simulink model "ACC_Scenario_006_cs"  (R2014b)
settings: Solver=ode5  SolverMode=SingleTasking  StartTime=0.0  StopTime=inf  FixedStep=1/100  RelTol=1e-3
PreLoadFcn:
  | mbxruntime.callbacks.PreLoadFcn(bdroot);
  | check_NUTS_defined;
  | 
  | assignin('base',['model_closed_' bdroot],false);addpath('../includes_ACC');
PostLoadFcn:
  | mbxruntime.callbacks.PostLoadFcn(bdroot);
InitFcn:
  | mbxruntime.callbacks.InitFcn(bdroot);
StartFcn:
  | mbxruntime.callbacks.StartFcn(bdroot);
StopFcn:
  | mbxruntime.callbacks.StopFcn(bdroot);
model workspace: external: MAT-File .\ACC_Scenario_006_cs_hws.mat (data not in the file)
undefined symbols (not defined in the file or in its folder): mbxruntime, OrientationPitch, OrientationRoll, PositionX, PositionY, PositionZ, tabledata, warningInitialVelocity, x0
undefined symbols (not defined in the file): ACC_Scenario_006_cs_061450488d6753c4, ACC_Scenario_006_cs_13896134c615b72a, ACC_Scenario_006_cs_18eaf2a52f2ef75d, ACC_Scenario_006_cs_59e375456829d2f0, ACC_Scenario_006_cs_8a2109b915871f11, ACC_Scenario_006_cs_a4f79cab717c06e2, ACC_Scenario_006_cs_Audi_A8_1_Dynamics_Simple_initialPitch, ACC_Scenario_006_cs_Audi_A8_1_Dynamics_Simple_initialRoll, ACC_Scenario_006_cs_Audi_A8_1_Dynamics_Simple_initialX, ACC_Scenario_006_cs_Audi_A8_1_Dynamics_Simple_initialY, ACC_Scenario_006_cs_Audi_A8_1_Dynamics_Simple_initialYaw, ACC_Scenario_006_cs_Audi_A8_1_Dynamics_Simple_initialZ, ACC_Scenario_006_cs_BMW_X5_1_Path_pathUniqueID, ACC_Scenario_006_cs_BMW_X5_1_SpeedProfile_speedProfileUniqueID, ACC_Scenario_006_cs_e4633c18fd34a832, ACC_Scenario_006_cs_f83c81dc10cd364a, ACC_Scenario_006_cs_Fiat_Bravo_1_Path_pathUniqueID, ACC_Scenario_006_cs_Ford_Fiesta_1_Path_pathUniqueID, ACC_Scenario_006_cs_Honda_Pan_European_1_Path_pathUniqueID, ACC_Scenario_006_cs_Mazda_RX8_1_Path_pathUniqueID, ACC_Scenario_006_cs_Sphere_1_Dynamics_Empty_STATE_Sphere_1_x0, ACC_Scenario_006_cs_Sphere_1_Dynamics_Empty_STATE_Sphere_1_y0, ACC_Scenario_006_cs_Sphere_1_Dynamics_Empty_STATE_Sphere_1_Yaw0, ACC_Scenario_006_cs_Sphere_1_Dynamics_Empty_STATE_Sphere_1_z0, ACC_Scenario_006_cs_Toyota_Yaris_1_Path_pathUniqueID, SteeringColumn, SteeringWheel, Wheel0, Wheel0_Suspension, Wheel1, Wheel1_Suspension, WheelL0, WheelL1, WheelR0, WheelR1
libraries: simulink_extras x60, simulink x21, PreScanSimulinkLibrary x5, PreScanUsefulBlocks x2
(part 13 of 24)

== system ACC_Scenario_006_cs/HighwayOverhang_10/VISUMatrixSign_Mux ==
  InformationPlate_15 : Inport
  InformationPlate_16 : Inport  Port=2
  InformationPlate_15_Conversion : DataTypeConversion
  InformationPlate_15_InitialResource : Constant  Value=5
  InformationPlate_15_Switch : Switch  Criteria=u2 ~= 0
  InformationPlate_16_Conversion : DataTypeConversion
  InformationPlate_16_InitialResource : Constant  Value=5
  InformationPlate_16_Switch : Switch  Criteria=u2 ~= 0
  SubMuxMatrixSign : Mux  Inputs=2
  MatrixSigns : Outport
  wires:
  SubMuxMatrixSign/1 -> MatrixSigns/1
  InformationPlate_15/1 -> InformationPlate_15_Switch/1, InformationPlate_15_Switch/2
  InformationPlate_15_InitialResource/1 -> InformationPlate_15_Switch/3
  InformationPlate_15_Switch/1 -> InformationPlate_15_Conversion/1
  InformationPlate_15_Conversion/1 -> SubMuxMatrixSign/1
  InformationPlate_16/1 -> InformationPlate_16_Switch/1, InformationPlate_16_Switch/2
  InformationPlate_16_InitialResource/1 -> InformationPlate_16_Switch/3
  InformationPlate_16_Switch/1 -> InformationPlate_16_Conversion/1
  InformationPlate_16_Conversion/1 -> SubMuxMatrixSign/2

== system ACC_Scenario_006_cs/HighwayOverhang_11/VISUMatrixSignLights_Mux ==
  MatrixSign_7 : Inport  Tag=inport/MatrixSign_7  PortDimensions=4  SampleTime=1/100  BusOutputAsStruct=on
  MatrixSign_8 : Inport  Tag=inport/MatrixSign_8  Port=2  PortDimensions=4  SampleTime=1/100  BusOutputAsStruct=on
  MuxVisuLights : Mux  Inputs=2
  VISUMatrixSignLights_HighwayOverhang_11 : Outport  Tag=outport/VisuMatrixSignLights  SampleTime=1/100
  wires:
  MuxVisuLights/1 -> VISUMatrixSignLights_HighwayOverhang_11/1
  MatrixSign_7/1 -> MuxVisuLights/1
  MatrixSign_8/1 -> MuxVisuLights/2

== system ACC_Scenario_006_cs/HighwayOverhang_11/VISUMatrixSign_Mux ==
  MatrixSign_7 : Inport
  MatrixSign_8 : Inport  Port=2
  MatrixSign_7_Conversion : DataTypeConversion
  MatrixSign_7_InitialResource : Constant
  MatrixSign_7_Switch : Switch  Criteria=u2 ~= 0
  MatrixSign_8_Conversion : DataTypeConversion
  MatrixSign_8_InitialResource : Constant
  MatrixSign_8_Switch : Switch  Criteria=u2 ~= 0
  SubMuxMatrixSign : Mux  Inputs=2
  MatrixSigns : Outport
  wires:
  SubMuxMatrixSign/1 -> MatrixSigns/1
  MatrixSign_7/1 -> MatrixSign_7_Switch/1, MatrixSign_7_Switch/2
  MatrixSign_7_InitialResource/1 -> MatrixSign_7_Switch/3
  MatrixSign_7_Switch/1 -> MatrixSign_7_Conversion/1
  MatrixSign_7_Conversion/1 -> SubMuxMatrixSign/1
  MatrixSign_8/1 -> MatrixSign_8_Switch/1, MatrixSign_8_Switch/2
  MatrixSign_8_InitialResource/1 -> MatrixSign_8_Switch/3
  MatrixSign_8_Switch/1 -> MatrixSign_8_Conversion/1
  MatrixSign_8_Conversion/1 -> SubMuxMatrixSign/2

== system ACC_Scenario_006_cs/HighwayOverhang_12/VISUMatrixSignLights_Mux ==
  MatrixSign_5 : Inport  Tag=inport/MatrixSign_5  PortDimensions=4  SampleTime=1/100  BusOutputAsStruct=on
  MatrixSign_6 : Inport  Tag=inport/MatrixSign_6  Port=2  PortDimensions=4  SampleTime=1/100  BusOutputAsStruct=on
  MuxVisuLights : Mux  Inputs=2
  VISUMatrixSignLights_HighwayOverhang_12 : Outport  Tag=outport/VisuMatrixSignLights  SampleTime=1/100
  wires:
  MuxVisuLights/1 -> VISUMatrixSignLights_HighwayOverhang_12/1
  MatrixSign_5/1 -> MuxVisuLights/1
  MatrixSign_6/1 -> MuxVisuLights/2

== system ACC_Scenario_006_cs/HighwayOverhang_12/VISUMatrixSign_Mux ==
  MatrixSign_5 : Inport
  MatrixSign_6 : Inport  Port=2
  MatrixSign_5_Conversion : DataTypeConversion
  MatrixSign_5_InitialResource : Constant
  MatrixSign_5_Switch : Switch  Criteria=u2 ~= 0
  MatrixSign_6_Conversion : DataTypeConversion
  MatrixSign_6_InitialResource : Constant
  MatrixSign_6_Switch : Switch  Criteria=u2 ~= 0
  SubMuxMatrixSign : Mux  Inputs=2
  MatrixSigns : Outport
  wires:
  SubMuxMatrixSign/1 -> MatrixSigns/1
  MatrixSign_5/1 -> MatrixSign_5_Switch/1, MatrixSign_5_Switch/2
  MatrixSign_5_InitialResource/1 -> MatrixSign_5_Switch/3
  MatrixSign_5_Switch/1 -> MatrixSign_5_Conversion/1
  MatrixSign_5_Conversion/1 -> SubMuxMatrixSign/1
  MatrixSign_6/1 -> MatrixSign_6_Switch/1, MatrixSign_6_Switch/2
  MatrixSign_6_InitialResource/1 -> MatrixSign_6_Switch/3
  MatrixSign_6_Switch/1 -> MatrixSign_6_Conversion/1
  MatrixSign_6_Conversion/1 -> SubMuxMatrixSign/2

== system ACC_Scenario_006_cs/HighwayOverhang_2/VISUMatrixSignLights_Mux ==
  MatrixSign_3 : Inport  Tag=inport/MatrixSign_3  PortDimensions=4  SampleTime=1/100  BusOutputAsStruct=on
  MatrixSign_4 : Inport  Tag=inport/MatrixSign_4  Port=2  PortDimensions=4  SampleTime=1/100  BusOutputAsStruct=on
  MuxVisuLights : Mux  Inputs=2
  VISUMatrixSignLights_HighwayOverhang_2 : Outport  Tag=outport/VisuMatrixSignLights  SampleTime=1/100
  wires:
  MuxVisuLights/1 -> VISUMatrixSignLights_HighwayOverhang_2/1
  MatrixSign_3/1 -> MuxVisuLights/1
  MatrixSign_4/1 -> MuxVisuLights/2

== system ACC_Scenario_006_cs/HighwayOverhang_2/VISUMatrixSign_Mux ==
  MatrixSign_3 : Inport
  MatrixSign_4 : Inport  Port=2
  MatrixSign_3_Conversion : DataTypeConversion
  MatrixSign_3_InitialResource : Constant
  MatrixSign_3_Switch : Switch  Criteria=u2 ~= 0
  MatrixSign_4_Conversion : DataTypeConversion
  MatrixSign_4_InitialResource : Constant
  MatrixSign_4_Switch : Switch  Criteria=u2 ~= 0
  SubMuxMatrixSign : Mux  Inputs=2
  MatrixSigns : Outport
  wires:
  SubMuxMatrixSign/1 -> MatrixSigns/1
  MatrixSign_3/1 -> MatrixSign_3_Switch/1, MatrixSign_3_Switch/2
  MatrixSign_3_InitialResource/1 -> MatrixSign_3_Switch/3
  MatrixSign_3_Switch/1 -> MatrixSign_3_Conversion/1
  MatrixSign_3_Conversion/1 -> SubMuxMatrixSign/1
  MatrixSign_4/1 -> MatrixSign_4_Switch/1, MatrixSign_4_Switch/2
  MatrixSign_4_InitialResource/1 -> MatrixSign_4_Switch/3
  MatrixSign_4_Switch/1 -> MatrixSign_4_Conversion/1
  MatrixSign_4_Conversion/1 -> SubMuxMatrixSign/2

== system ACC_Scenario_006_cs/HighwayOverhang_3/VISUMatrixSign_Mux ==
  InformationPlate_1 : Inport
  InformationPlate_2 : Inport  Port=2
  InformationPlate_1_Conversion : DataTypeConversion
  InformationPlate_1_InitialResource : Constant  Value=2
  InformationPlate_1_Switch : Switch  Criteria=u2 ~= 0
  InformationPlate_2_Conversion : DataTypeConversion
  InformationPlate_2_InitialResource : Constant  Value=2
  InformationPlate_2_Switch : Switch  Criteria=u2 ~= 0
  SubMuxMatrixSign : Mux  Inputs=2
  MatrixSigns : Outport
  wires:
  SubMuxMatrixSign/1 -> MatrixSigns/1
  InformationPlate_1/1 -> InformationPlate_1_Switch/1, InformationPlate_1_Switch/2
  InformationPlate_1_InitialResource/1 -> InformationPlate_1_Switch/3
  InformationPlate_1_Switch/1 -> InformationPlate_1_Conversion/1
  InformationPlate_1_Conversion/1 -> SubMuxMatrixSign/1
  InformationPlate_2/1 -> InformationPlate_2_Switch/1, InformationPlate_2_Switch/2
  InformationPlate_2_InitialResource/1 -> InformationPlate_2_Switch/3
  InformationPlate_2_Switch/1 -> InformationPlate_2_Conversion/1
  InformationPlate_2_Conversion/1 -> SubMuxMatrixSign/2

== system ACC_Scenario_006_cs/HighwayOverhang_4/VISUMatrixSign_Mux ==
  InformationPlate_3 : Inport
  InformationPlate_4 : Inport  Port=2
  InformationPlate_3_Conversion : DataTypeConversion
  InformationPlate_3_InitialResource : Constant  Value=2
  InformationPlate_3_Switch : Switch  Criteria=u2 ~= 0
  InformationPlate_4_Conversion : DataTypeConversion
  InformationPlate_4_InitialResource : Constant  Value=2
  InformationPlate_4_Switch : Switch  Criteria=u2 ~= 0
  SubMuxMatrixSign : Mux  Inputs=2
  MatrixSigns : Outport
  wires:
  SubMuxMatrixSign/1 -> MatrixSigns/1
  InformationPlate_3/1 -> InformationPlate_3_Switch/1, InformationPlate_3_Switch/2
  InformationPlate_3_InitialResource/1 -> InformationPlate_3_Switch/3
  InformationPlate_3_Switch/1 -> InformationPlate_3_Conversion/1
  InformationPlate_3_Conversion/1 -> SubMuxMatrixSign/1
  InformationPlate_4/1 -> InformationPlate_4_Switch/1, InformationPlate_4_Switch/2
  InformationPlate_4_InitialResource/1 -> InformationPlate_4_Switch/3
  InformationPlate_4_Switch/1 -> InformationPlate_4_Conversion/1
  InformationPlate_4_Conversion/1 -> SubMuxMatrixSign/2

== system ACC_Scenario_006_cs/HighwayOverhang_5/VISUMatrixSign_Mux ==
  InformationPlate_5 : Inport
  InformationPlate_6 : Inport  Port=2
  InformationPlate_5_Conversion : DataTypeConversion
  InformationPlate_5_InitialResource : Constant  Value=3
  InformationPlate_5_Switch : Switch  Criteria=u2 ~= 0
  InformationPlate_6_Conversion : DataTypeConversion
  InformationPlate_6_InitialResource : Constant  Value=3
  InformationPlate_6_Switch : Switch  Criteria=u2 ~= 0
  SubMuxMatrixSign : Mux  Inputs=2
  MatrixSigns : Outport
  wires:
  SubMuxMatrixSign/1 -> MatrixSigns/1
  InformationPlate_5/1 -> InformationPlate_5_Switch/1, InformationPlate_5_Switch/2
  InformationPlate_5_InitialResource/1 -> InformationPlate_5_Switch/3
  InformationPlate_5_Switch/1 -> InformationPlate_5_Conversion/1
  InformationPlate_5_Conversion/1 -> SubMuxMatrixSign/1
  InformationPlate_6/1 -> InformationPlate_6_Switch/1, InformationPlate_6_Switch/2
  InformationPlate_6_InitialResource/1 -> InformationPlate_6_Switch/3
  InformationPlate_6_Switch/1 -> InformationPlate_6_Conversion/1
  InformationPlate_6_Conversion/1 -> SubMuxMatrixSign/2

== system ACC_Scenario_006_cs/HighwayOverhang_6/VISUMatrixSign_Mux ==
  InformationPlate_7 : Inport
  InformationPlate_8 : Inport  Port=2
  InformationPlate_7_Conversion : DataTypeConversion
  InformationPlate_7_InitialResource : Constant  Value=3
  InformationPlate_7_Switch : Switch  Criteria=u2 ~= 0
  InformationPlate_8_Conversion : DataTypeConversion
  InformationPlate_8_InitialResource : Constant  Value=3
  InformationPlate_8_Switch : Switch  Criteria=u2 ~= 0
  SubMuxMatrixSign : Mux  Inputs=2
  MatrixSigns : Outport
  wires:
  SubMuxMatrixSign/1 -> MatrixSigns/1
  InformationPlate_7/1 -> InformationPlate_7_Switch/1, InformationPlate_7_Switch/2
  InformationPlate_7_InitialResource/1 -> InformationPlate_7_Switch/3
  InformationPlate_7_Switch/1 -> InformationPlate_7_Conversion/1
  InformationPlate_7_Conversion/1 -> SubMuxMatrixSign/1
  InformationPlate_8/1 -> InformationPlate_8_Switch/1, InformationPlate_8_Switch/2
  InformationPlate_8_InitialResource/1 -> InformationPlate_8_Switch/3
  InformationPlate_8_Switch/1 -> InformationPlate_8_Conversion/1
  InformationPlate_8_Conversion/1 -> SubMuxMatrixSign/2

== system ACC_Scenario_006_cs/HighwayOverhang_7/VISUMatrixSign_Mux ==
  InformationPlate_9 : Inport
  InformationPlate_10 : Inport  Port=2
  InformationPlate_10_Conversion : DataTypeConversion
  InformationPlate_10_InitialResource : Constant  Value=4
  InformationPlate_10_Switch : Switch  Criteria=u2 ~= 0
  InformationPlate_9_Conversion : DataTypeConversion
  InformationPlate_9_InitialResource : Constant  Value=4
  InformationPlate_9_Switch : Switch  Criteria=u2 ~= 0
  SubMuxMatrixSign : Mux  Inputs=2
  MatrixSigns : Outport
  wires:
  SubMuxMatrixSign/1 -> MatrixSigns/1
  InformationPlate_9/1 -> InformationPlate_9_Switch/1, InformationPlate_9_Switch/2
  InformationPlate_9_InitialResource/1 -> InformationPlate_9_Switch/3
  InformationPlate_9_Switch/1 -> InformationPlate_9_Conversion/1
  InformationPlate_9_Conversion/1 -> SubMuxMatrixSign/1
  InformationPlate_10/1 -> InformationPlate_10_Switch/1, InformationPlate_10_Switch/2
  InformationPlate_10_InitialResource/1 -> InformationPlate_10_Switch/3
  InformationPlate_10_Switch/1 -> InformationPlate_10_Conversion/1
  InformationPlate_10_Conversion/1 -> SubMuxMatrixSign/2

== system ACC_Scenario_006_cs/HighwayOverhang_8/VISUMatrixSign_Mux ==
  InformationPlate_11 : Inport
  InformationPlate_12 : Inport  Port=2
  InformationPlate_11_Conversion : DataTypeConversion
  InformationPlate_11_InitialResource : Constant  Value=4
  InformationPlate_11_Switch : Switch  Criteria=u2 ~= 0
  InformationPlate_12_Conversion : DataTypeConversion
  InformationPlate_12_InitialResource : Constant  Value=4
  InformationPlate_12_Switch : Switch  Criteria=u2 ~= 0
  SubMuxMatrixSign : Mux  Inputs=2
  MatrixSigns : Outport
  wires:
  SubMuxMatrixSign/1 -> MatrixSigns/1
  InformationPlate_11/1 -> InformationPlate_11_Switch/1, InformationPlate_11_Switch/2
  InformationPlate_11_InitialResource/1 -> InformationPlate_11_Switch/3
  InformationPlate_11_Switch/1 -> InformationPlate_11_Conversion/1
  InformationPlate_11_Conversion/1 -> SubMuxMatrixSign/1
  InformationPlate_12/1 -> InformationPlate_12_Switch/1, InformationPlate_12_Switch/2
  InformationPlate_12_InitialResource/1 -> InformationPlate_12_Switch/3
  InformationPlate_12_Switch/1 -> InformationPlate_12_Conversion/1
  InformationPlate_12_Conversion/1 -> SubMuxMatrixSign/2

== system ACC_Scenario_006_cs/HighwayOverhang_9/VISUMatrixSign_Mux ==
  InformationPlate_13 : Inport
  InformationPlate_14 : Inport  Port=2
  InformationPlate_13_Conversion : DataTypeConversion
  InformationPlate_13_InitialResource : Constant  Value=5
  InformationPlate_13_Switch : Switch  Criteria=u2 ~= 0
  InformationPlate_14_Conversion : DataTypeConversion
  InformationPlate_14_InitialResource : Constant  Value=5
  InformationPlate_14_Switch : Switch  Criteria=u2 ~= 0
  SubMuxMatrixSign : Mux  Inputs=2
  MatrixSigns : Outport
  wires:
  SubMuxMatrixSign/1 -> MatrixSigns/1
  InformationPlate_13/1 -> InformationPlate_13_Switch/1, InformationPlate_13_Switch/2
  InformationPlate_13_InitialResource/1 -> InformationPlate_13_Switch/3
  InformationPlate_13_Switch/1 -> InformationPlate_13_Conversion/1
  InformationPlate_13_Conversion/1 -> SubMuxMatrixSign/1
  InformationPlate_14/1 -> InformationPlate_14_Switch/1, InformationPlate_14_Switch/2
  InformationPlate_14_InitialResource/1 -> InformationPlate_14_Switch/3
  InformationPlate_14_Switch/1 -> InformationPlate_14_Conversion/1
  InformationPlate_14_Conversion/1 -> SubMuxMatrixSign/2

== system ACC_Scenario_006_cs/Honda_Pan_European_1/Brake_light_center_Mux ==
  MSCD [Cd] : Inport
  Position (xyz) [m] : Inport  Port=2
  Orientation (RPY) [deg] : Inport  Port=3
  Color [-] : Inport  Port=4
  TextureResourceID [-] : Inport  Port=5
  Bus Creator : BusCreator  Inputs='Intensity','Position','Orientation','Color','TextureResourceID'  OutDataTypeStr=Bus: PRESCAN_VISULIGHTACTUATOR_DATA  NonVirtualBus=on
  Bus Creator1 : BusCreator  Inputs=3  OutDataTypeStr=Bus: PRESCAN_RGB_DATA  NonVirtualBus=on
  Bus Creator2 : BusCreator  Inputs=3  OutDataTypeStr=Bus: PRESCAN_RPY_DATA  NonVirtualBus=on
  Bus Creator3 : BusCreator  Inputs=3  OutDataTypeStr=Bus: PRESCAN_XYZ_DATA  NonVirtualBus=on
  Data Type Conversion : DataTypeConversion  OutDataTypeStr=int32  RndMeth=Nearest
  Degrees to Radians : simulink_extras/Transformations/Degrees to Radians
  Demux : Demux  Outputs=3
  Demux1 : Demux  Outputs=3
  Demux2 : Demux  Outputs=3
  Lights : Outport
  wires:
  TextureResourceID [-]/1 -> Data Type Conversion/1  "TextureResourceID"
  MSCD [Cd]/1 -> Bus Creator/1  "Intensity"
  Bus Creator/1 -> Lights/1
  Demux/1 -> Bus Creator1/1  "R"
  Demux/2 -> Bus Creator1/2  "G"
  Demux/3 -> Bus Creator1/3  "B"
  Color [-]/1 -> Demux/1  "Color"
  Bus Creator1/1 -> Bus Creator/4  "Color"
  Demux1/1 -> Bus Creator2/1  "Roll"
  Demux1/2 -> Bus Creator2/2  "Pitch"
  Demux1/3 -> Bus Creator2/3  "Yaw"
  Orientation (RPY) [deg]/1 -> Degrees to Radians/1  "Orientation"
  Bus Creator2/1 -> Bus Creator/3  "Orientation"
  Demux2/1 -> Bus Creator3/1  "X"
  Demux2/2 -> Bus Creator3/2  "Y"
  Demux2/3 -> Bus Creator3/3  "Z"
  Position (xyz) [m]/1 -> Demux2/1  "Position"
  Bus Creator3/1 -> Bus Creator/2  "Position"
  Data Type Conversion/1 -> Bus Creator/5  "TextureResourceID"
  Degrees to Radians/1 -> Demux1/1

== system ACC_Scenario_006_cs/Honda_Pan_European_1/Indicator_front_left_Mux ==
  MSCD [Cd] : Inport
  Position (xyz) [m] : Inport  Port=2
  Orientation (RPY) [deg] : Inport  Port=3
  Color [-] : Inport  Port=4
  TextureResourceID [-] : Inport  Port=5
  Bus Creator : BusCreator  Inputs='Intensity','Position','Orientation','Color','TextureResourceID'  OutDataTypeStr=Bus: PRESCAN_VISULIGHTACTUATOR_DATA  NonVirtualBus=on
  Bus Creator1 : BusCreator  Inputs=3  OutDataTypeStr=Bus: PRESCAN_RGB_DATA  NonVirtualBus=on
  Bus Creator2 : BusCreator  Inputs=3  OutDataTypeStr=Bus: PRESCAN_RPY_DATA  NonVirtualBus=on
  Bus Creator3 : BusCreator  Inputs=3  OutDataTypeStr=Bus: PRESCAN_XYZ_DATA  NonVirtualBus=on
  Data Type Conversion : DataTypeConversion  OutDataTypeStr=int32  RndMeth=Nearest
  Degrees to Radians : simulink_extras/Transformations/Degrees to Radians
  Demux : Demux  Outputs=3
  Demux1 : Demux  Outputs=3
  Demux2 : Demux  Outputs=3
  Lights : Outport
  wires:
  TextureResourceID [-]/1 -> Data Type Conversion/1  "TextureResourceID"
  MSCD [Cd]/1 -> Bus Creator/1  "Intensity"
  Bus Creator/1 -> Lights/1
  Demux/1 -> Bus Creator1/1  "R"
  Demux/2 -> Bus Creator1/2  "G"
  Demux/3 -> Bus Creator1/3  "B"
  Color [-]/1 -> Demux/1  "Color"
  Bus Creator1/1 -> Bus Creator/4  "Color"
  Demux1/1 -> Bus Creator2/1  "Roll"
  Demux1/2 -> Bus Creator2/2  "Pitch"
  Demux1/3 -> Bus Creator2/3  "Yaw"
  Orientation (RPY) [deg]/1 -> Degrees to Radians/1  "Orientation"
  Bus Creator2/1 -> Bus Creator/3  "Orientation"
  Demux2/1 -> Bus Creator3/1  "X"
  Demux2/2 -> Bus Creator3/2  "Y"
  Demux2/3 -> Bus Creator3/3  "Z"
  Position (xyz) [m]/1 -> Demux2/1  "Position"
  Bus Creator3/1 -> Bus Creator/2  "Position"
  Data Type Conversion/1 -> Bus Creator/5  "TextureResourceID"
  Degrees to Radians/1 -> Demux1/1

== system ACC_Scenario_006_cs/Honda_Pan_European_1/Indicator_front_right_Mux ==
  MSCD [Cd] : Inport
  Position (xyz) [m] : Inport  Port=2
  Orientation (RPY) [deg] : Inport  Port=3
  Color [-] : Inport  Port=4
  TextureResourceID [-] : Inport  Port=5
  Bus Creator : BusCreator  Inputs='Intensity','Position','Orientation','Color','TextureResourceID'  OutDataTypeStr=Bus: PRESCAN_VISULIGHTACTUATOR_DATA  NonVirtualBus=on
  Bus Creator1 : BusCreator  Inputs=3  OutDataTypeStr=Bus: PRESCAN_RGB_DATA  NonVirtualBus=on
  Bus Creator2 : BusCreator  Inputs=3  OutDataTypeStr=Bus: PRESCAN_RPY_DATA  NonVirtualBus=on
  Bus Creator3 : BusCreator  Inputs=3  OutDataTypeStr=Bus: PRESCAN_XYZ_DATA  NonVirtualBus=on
  Data Type Conversion : DataTypeConversion  OutDataTypeStr=int32  RndMeth=Nearest
  Degrees to Radians : simulink_extras/Transformations/Degrees to Radians
  Demux : Demux  Outputs=3
  Demux1 : Demux  Outputs=3
  Demux2 : Demux  Outputs=3
  Lights : Outport
  wires:
  TextureResourceID [-]/1 -> Data Type Conversion/1  "TextureResourceID"
  MSCD [Cd]/1 -> Bus Creator/1  "Intensity"
  Bus Creator/1 -> Lights/1
  Demux/1 -> Bus Creator1/1  "R"
  Demux/2 -> Bus Creator1/2  "G"
  Demux/3 -> Bus Creator1/3  "B"
  Color [-]/1 -> Demux/1  "Color"
  Bus Creator1/1 -> Bus Creator/4  "Color"
  Demux1/1 -> Bus Creator2/1  "Roll"
  Demux1/2 -> Bus Creator2/2  "Pitch"
  Demux1/3 -> Bus Creator2/3  "Yaw"
  Orientation (RPY) [deg]/1 -> Degrees to Radians/1  "Orientation"
  Bus Creator2/1 -> Bus Creator/3  "Orientation"
  Demux2/1 -> Bus Creator3/1  "X"
  Demux2/2 -> Bus Creator3/2  "Y"
  Demux2/3 -> Bus Creator3/3  "Z"
  Position (xyz) [m]/1 -> Demux2/1  "Position"
  Bus Creator3/1 -> Bus Creator/2  "Position"
  Data Type Conversion/1 -> Bus Creator/5  "TextureResourceID"
  Degrees to Radians/1 -> Demux1/1

== system ACC_Scenario_006_cs/Honda_Pan_European_1/Indicator_rear_left_Mux ==
  MSCD [Cd] : Inport
  Position (xyz) [m] : Inport  Port=2
  Orientation (RPY) [deg] : Inport  Port=3
  Color [-] : Inport  Port=4
  TextureResourceID [-] : Inport  Port=5
  Bus Creator : BusCreator  Inputs='Intensity','Position','Orientation','Color','TextureResourceID'  OutDataTypeStr=Bus: PRESCAN_VISULIGHTACTUATOR_DATA  NonVirtualBus=on
  Bus Creator1 : BusCreator  Inputs=3  OutDataTypeStr=Bus: PRESCAN_RGB_DATA  NonVirtualBus=on
  Bus Creator2 : BusCreator  Inputs=3  OutDataTypeStr=Bus: PRESCAN_RPY_DATA  NonVirtualBus=on
  Bus Creator3 : BusCreator  Inputs=3  OutDataTypeStr=Bus: PRESCAN_XYZ_DATA  NonVirtualBus=on
  Data Type Conversion : DataTypeConversion  OutDataTypeStr=int32  RndMeth=Nearest
  Degrees to Radians : simulink_extras/Transformations/Degrees to Radians
  Demux : Demux  Outputs=3
  Demux1 : Demux  Outputs=3
  Demux2 : Demux  Outputs=3
  Lights : Outport
  wires:
  TextureResourceID [-]/1 -> Data Type Conversion/1  "TextureResourceID"
  MSCD [Cd]/1 -> Bus Creator/1  "Intensity"
  Bus Creator/1 -> Lights/1
  Demux/1 -> Bus Creator1/1  "R"
  Demux/2 -> Bus Creator1/2  "G"
  Demux/3 -> Bus Creator1/3  "B"
  Color [-]/1 -> Demux/1  "Color"
  Bus Creator1/1 -> Bus Creator/4  "Color"
  Demux1/1 -> Bus Creator2/1  "Roll"
  Demux1/2 -> Bus Creator2/2  "Pitch"
  Demux1/3 -> Bus Creator2/3  "Yaw"
  Orientation (RPY) [deg]/1 -> Degrees to Radians/1  "Orientation"
  Bus Creator2/1 -> Bus Creator/3  "Orientation"
  Demux2/1 -> Bus Creator3/1  "X"
  Demux2/2 -> Bus Creator3/2  "Y"
  Demux2/3 -> Bus Creator3/3  "Z"
  Position (xyz) [m]/1 -> Demux2/1  "Position"
  Bus Creator3/1 -> Bus Creator/2  "Position"
  Data Type Conversion/1 -> Bus Creator/5  "TextureResourceID"
  Degrees to Radians/1 -> Demux1/1

== system ACC_Scenario_006_cs/Honda_Pan_European_1/Indicator_rear_right_Mux ==
  MSCD [Cd] : Inport
  Position (xyz) [m] : Inport  Port=2
  Orientation (RPY) [deg] : Inport  Port=3
  Color [-] : Inport  Port=4
  TextureResourceID [-] : Inport  Port=5
  Bus Creator : BusCreator  Inputs='Intensity','Position','Orientation','Color','TextureResourceID'  OutDataTypeStr=Bus: PRESCAN_VISULIGHTACTUATOR_DATA  NonVirtualBus=on
  Bus Creator1 : BusCreator  Inputs=3  OutDataTypeStr=Bus: PRESCAN_RGB_DATA  NonVirtualBus=on
  Bus Creator2 : BusCreator  Inputs=3  OutDataTypeStr=Bus: PRESCAN_RPY_DATA  NonVirtualBus=on
  Bus Creator3 : BusCreator  Inputs=3  OutDataTypeStr=Bus: PRESCAN_XYZ_DATA  NonVirtualBus=on
  Data Type Conversion : DataTypeConversion  OutDataTypeStr=int32  RndMeth=Nearest
  Degrees to Radians : simulink_extras/Transformations/Degrees to Radians
  Demux : Demux  Outputs=3
  Demux1 : Demux  Outputs=3
  Demux2 : Demux  Outputs=3
  Lights : Outport
  wires:
  TextureResourceID [-]/1 -> Data Type Conversion/1  "TextureResourceID"
  MSCD [Cd]/1 -> Bus Creator/1  "Intensity"
  Bus Creator/1 -> Lights/1
  Demux/1 -> Bus Creator1/1  "R"
  Demux/2 -> Bus Creator1/2  "G"
  Demux/3 -> Bus Creator1/3  "B"
  Color [-]/1 -> Demux/1  "Color"
  Bus Creator1/1 -> Bus Creator/4  "Color"
  Demux1/1 -> Bus Creator2/1  "Roll"
  Demux1/2 -> Bus Creator2/2  "Pitch"
  Demux1/3 -> Bus Creator2/3  "Yaw"
  Orientation (RPY) [deg]/1 -> Degrees to Radians/1  "Orientation"
  Bus Creator2/1 -> Bus Creator/3  "Orientation"
  Demux2/1 -> Bus Creator3/1  "X"
  Demux2/2 -> Bus Creator3/2  "Y"
  Demux2/3 -> Bus Creator3/3  "Z"
  Position (xyz) [m]/1 -> Demux2/1  "Position"
  Bus Creator3/1 -> Bus Creator/2  "Position"
  Data Type Conversion/1 -> Bus Creator/5  "TextureResourceID"
  Degrees to Radians/1 -> Demux1/1

== system ACC_Scenario_006_cs/Honda_Pan_European_1/SELF_Demux ==
  SELF : Inport  OutDataTypeStr=Bus: PRESCAN_SELFSENSORDATA
  Bus Selector : BusSelector  OutputSignals=PositionX,PositionY,PositionZ,OrientationRoll,OrientationPitch,OrientationYaw,Velocity,Yaw_rate,Lat,Long,Alt
  Demux2 : Demux  Outputs=3
  Gain : Gain  Gain=180/pi
  Gain1 : Gain  Gain=180/pi
  Vector Concatenate1 : Concatenate  NumInputs=3
  compas converter : Subsystem
  x [m] : Outport
  y [m] : Outport  Port=2
  z [m] : Outport  Port=3
  rotx [deg] : Outport  Port=4
  roty [deg] : Outport  Port=5
  rotz [deg] : Outport  Port=6
  GPS lat [deg] : Outport  Port=7
  GPS long [deg] : Outport  Port=8
  GPS alt [m] : Outport  Port=9
  velocity [m/s] : Outport  Port=10
  heading [deg] : Outport  Port=11
  yaw rate [deg/s] : Outport  Port=12
  wires:
  Bus Selector/11 -> GPS alt [m]/1  "<Alt>"
  Bus Selector/10 -> GPS long [deg]/1  "<Long>"
  Bus Selector/9 -> GPS lat [deg]/1  "<Lat>"
  Bus Selector/8 -> Gain1/1  "<Yaw_rate>"
  Bus Selector/7 -> velocity [m/s]/1  "<Velocity>"
  Bus Selector/6 -> compas converter/1(rotz [rad]), Vector Concatenate1/3  "<OrientationYaw>"
  Bus Selector/5 -> Vector Concatenate1/2  "<OrientationPitch>"
  Bus Selector/4 -> Vector Concatenate1/1  "<OrientationRoll>"
  Vector Concatenate1/1 -> Gain/1
  Bus Selector/3 -> z [m]/1  "<PositionZ>"
  Bus Selector/2 -> y [m]/1  "<PositionY>"
  Bus Selector/1 -> x [m]/1  "<PositionX>"
  SELF/1 -> Bus Selector/1
  Gain/1 -> Demux2/1
  Demux2/1 -> rotx [deg]/1
  Demux2/2 -> roty [deg]/1
  Demux2/3 -> rotz [deg]/1
  compas converter/1(heading [deg]) -> heading [deg]/1
  Gain1/1 -> yaw rate [deg/s]/1

== system ACC_Scenario_006_cs/Honda_Pan_European_1/V2R_WheelMC ==
  Velocity [m/s] : Inport  SampleTime=TimeStep
  Discrete-Time Integrator : DiscreteIntegrator  SampleTime=TimeStep
  omega=V/Rwheel : Gain  Gain=1/TireRadius
  Rotation [rad] : Outport
  wires:
  Velocity [m/s]/1 -> omega=V/Rwheel/1
  omega=V/Rwheel/1 -> Discrete-Time Integrator/1  "rotational speed [rad/s]"
  Discrete-Time Integrator/1 -> Rotation [rad]/1  "roty"

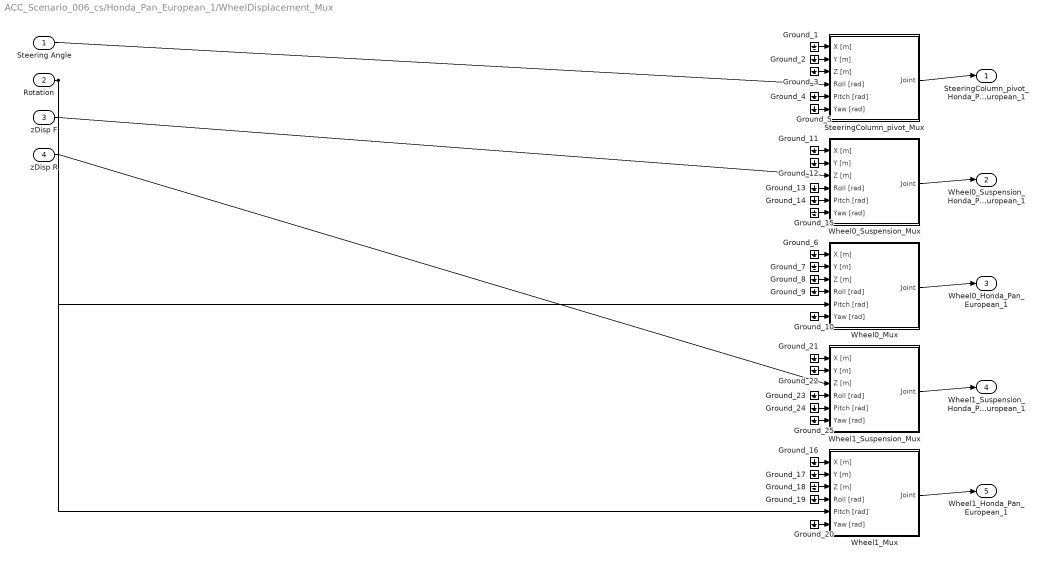
== system ACC_Scenario_006_cs/Honda_Pan_European_1/WheelDisplacement_Mux ==
  Steering Angle : Inport  Tag=inport/JointGroup  SampleTime=1/100  BusOutputAsStruct=on
  Rotation : Inport  Tag=inport/JointGroup  Port=2  SampleTime=1/100  BusOutputAsStruct=on
  zDisp F : Inport  Tag=inport/JointGroup  Port=3  SampleTime=1/100  BusOutputAsStruct=on
  zDisp R : Inport  Tag=inport/JointGroup  Port=4  SampleTime=1/100  BusOutputAsStruct=on
  Ground_{1..25} (25 alike) : Ground
  SteeringColumn_pivot_Mux : Subsystem  Tag=mux/Joint  mask(PreScan Mux Block){DisplayName=SteeringColumn}
      mask prompts: DisplayName "Display Name"
      mask help:
      | This block simulates a generic joint used for generic models. This joint can be enabled/disabled from the GUI.
      |
      | For more information, please click Help.
      settings: DeleteFcn=PreScanBlockDeleteFcn;
      mask Help: eval('openHelp(254)')
  Wheel0_Mux : Subsystem  Tag=mux/Joint  mask(PreScan Mux Block){DisplayName=Wheel0}
      mask prompts: DisplayName "Display Name"
      mask help:
      | This block simulates a generic joint used for generic models. This joint can be enabled/disabled from the GUI.
      |
      | For more information, please click Help.
      settings: DeleteFcn=PreScanBlockDeleteFcn;
      mask Help: eval('openHelp(254)')
  Wheel0_Suspension_Mux : Subsystem  Tag=mux/Joint  mask(PreScan Mux Block){DisplayName=Wheel0_Suspension}
      mask prompts: DisplayName "Display Name"
      mask help:
      | This block simulates a generic joint used for generic models. This joint can be enabled/disabled from the GUI.
      |
      | For more information, please click Help.
      settings: DeleteFcn=PreScanBlockDeleteFcn;
      mask Help: eval('openHelp(254)')
  Wheel1_Mux : Subsystem  Tag=mux/Joint  mask(PreScan Mux Block){DisplayName=Wheel1}
      mask prompts: DisplayName "Display Name"
      mask help:
      | This block simulates a generic joint used for generic models. This joint can be enabled/disabled from the GUI.
      |
      | For more information, please click Help.
      settings: DeleteFcn=PreScanBlockDeleteFcn;
      mask Help: eval('openHelp(254)')
  Wheel1_Suspension_Mux : Subsystem  Tag=mux/Joint  mask(PreScan Mux Block){DisplayName=Wheel1_Suspension}
      mask prompts: DisplayName "Display Name"
      mask help:
      | This block simulates a generic joint used for generic models. This joint can be enabled/disabled from the GUI.
      |
      | For more information, please click Help.
      settings: DeleteFcn=PreScanBlockDeleteFcn;
      mask Help: eval('openHelp(254)')
  SteeringColumn_pivot_Honda_Pan_European_1 : Outport  Tag=outport/JointActuator  OutDataTypeStr=Bus: PRESCAN_POSE_DATA  SampleTime=1/100
  Wheel0_Suspension_Honda_Pan_European_1 : Outport  Tag=outport/JointActuator  Port=2  OutDataTypeStr=Bus: PRESCAN_POSE_DATA  SampleTime=1/100
  Wheel0_Honda_Pan_European_1 : Outport  Tag=outport/JointActuator  Port=3  OutDataTypeStr=Bus: PRESCAN_POSE_DATA  SampleTime=1/100
  Wheel1_Suspension_Honda_Pan_European_1 : Outport  Tag=outport/JointActuator  Port=4  OutDataTypeStr=Bus: PRESCAN_POSE_DATA  SampleTime=1/100
  Wheel1_Honda_Pan_European_1 : Outport  Tag=outport/JointActuator  Port=5  OutDataTypeStr=Bus: PRESCAN_POSE_DATA  SampleTime=1/100
  wires:
  SteeringColumn_pivot_Mux/1(Joint) -> SteeringColumn_pivot_Honda_Pan_European_1/1
  Wheel0_Suspension_Mux/1(Joint) -> Wheel0_Suspension_Honda_Pan_European_1/1
  Wheel0_Mux/1(Joint) -> Wheel0_Honda_Pan_European_1/1
  Wheel1_Suspension_Mux/1(Joint) -> Wheel1_Suspension_Honda_Pan_European_1/1
  Wheel1_Mux/1(Joint) -> Wheel1_Honda_Pan_European_1/1
  Steering Angle/1 -> SteeringColumn_pivot_Mux/4(Roll [rad])
  Rotation/1 -> Wheel0_Mux/5(Pitch [rad]), Wheel1_Mux/5(Pitch [rad])
  zDisp F/1 -> Wheel0_Suspension_Mux/3(Z [m])
  zDisp R/1 -> Wheel1_Suspension_Mux/3(Z [m])
  Ground_1/1 -> SteeringColumn_pivot_Mux/1(X [m])
  Ground_2/1 -> SteeringColumn_pivot_Mux/2(Y [m])
  Ground_3/1 -> SteeringColumn_pivot_Mux/3(Z [m])
  Ground_4/1 -> SteeringColumn_pivot_Mux/5(Pitch [rad])
  Ground_5/1 -> SteeringColumn_pivot_Mux/6(Yaw [rad])
  Ground_6/1 -> Wheel0_Mux/1(X [m])
  Ground_7/1 -> Wheel0_Mux/2(Y [m])
  Ground_8/1 -> Wheel0_Mux/3(Z [m])
  Ground_9/1 -> Wheel0_Mux/4(Roll [rad])
  Ground_10/1 -> Wheel0_Mux/6(Yaw [rad])
  Ground_11/1 -> Wheel0_Suspension_Mux/1(X [m])
  Ground_12/1 -> Wheel0_Suspension_Mux/2(Y [m])
  Ground_13/1 -> Wheel0_Suspension_Mux/4(Roll [rad])
  Ground_14/1 -> Wheel0_Suspension_Mux/5(Pitch [rad])
  Ground_15/1 -> Wheel0_Suspension_Mux/6(Yaw [rad])
  Ground_16/1 -> Wheel1_Mux/1(X [m])
  Ground_17/1 -> Wheel1_Mux/2(Y [m])
  Ground_18/1 -> Wheel1_Mux/3(Z [m])
  Ground_19/1 -> Wheel1_Mux/4(Roll [rad])
  Ground_20/1 -> Wheel1_Mux/6(Yaw [rad])
  Ground_21/1 -> Wheel1_Suspension_Mux/1(X [m])
  Ground_22/1 -> Wheel1_Suspension_Mux/2(Y [m])
  Ground_23/1 -> Wheel1_Suspension_Mux/4(Roll [rad])
  Ground_24/1 -> Wheel1_Suspension_Mux/5(Pitch [rad])
  Ground_25/1 -> Wheel1_Suspension_Mux/6(Yaw [rad])

== system ACC_Scenario_006_cs/Mazda_RX8_1/Brake_light_center_Mux ==
  MSCD [Cd] : Inport
  Position (xyz) [m] : Inport  Port=2
  Orientation (RPY) [deg] : Inport  Port=3
  Color [-] : Inport  Port=4
  TextureResourceID [-] : Inport  Port=5
  Bus Creator : BusCreator  Inputs='Intensity','Position','Orientation','Color','TextureResourceID'  OutDataTypeStr=Bus: PRESCAN_VISULIGHTACTUATOR_DATA  NonVirtualBus=on
  Bus Creator1 : BusCreator  Inputs=3  OutDataTypeStr=Bus: PRESCAN_RGB_DATA  NonVirtualBus=on
  Bus Creator2 : BusCreator  Inputs=3  OutDataTypeStr=Bus: PRESCAN_RPY_DATA  NonVirtualBus=on
  Bus Creator3 : BusCreator  Inputs=3  OutDataTypeStr=Bus: PRESCAN_XYZ_DATA  NonVirtualBus=on
  Data Type Conversion : DataTypeConversion  OutDataTypeStr=int32  RndMeth=Nearest
  Degrees to Radians : simulink_extras/Transformations/Degrees to Radians
  Demux : Demux  Outputs=3
  Demux1 : Demux  Outputs=3
  Demux2 : Demux  Outputs=3
  Lights : Outport
  wires:
  TextureResourceID [-]/1 -> Data Type Conversion/1  "TextureResourceID"
  MSCD [Cd]/1 -> Bus Creator/1  "Intensity"
  Bus Creator/1 -> Lights/1
  Demux/1 -> Bus Creator1/1  "R"
  Demux/2 -> Bus Creator1/2  "G"
  Demux/3 -> Bus Creator1/3  "B"
  Color [-]/1 -> Demux/1  "Color"
  Bus Creator1/1 -> Bus Creator/4  "Color"
  Demux1/1 -> Bus Creator2/1  "Roll"
  Demux1/2 -> Bus Creator2/2  "Pitch"
  Demux1/3 -> Bus Creator2/3  "Yaw"
  Orientation (RPY) [deg]/1 -> Degrees to Radians/1  "Orientation"
  Bus Creator2/1 -> Bus Creator/3  "Orientation"
  Demux2/1 -> Bus Creator3/1  "X"
  Demux2/2 -> Bus Creator3/2  "Y"
  Demux2/3 -> Bus Creator3/3  "Z"
  Position (xyz) [m]/1 -> Demux2/1  "Position"
  Bus Creator3/1 -> Bus Creator/2  "Position"
  Data Type Conversion/1 -> Bus Creator/5  "TextureResourceID"
  Degrees to Radians/1 -> Demux1/1

== system ACC_Scenario_006_cs/Mazda_RX8_1/Brake_light_left_Mux ==
  MSCD [Cd] : Inport
  Position (xyz) [m] : Inport  Port=2
  Orientation (RPY) [deg] : Inport  Port=3
  Color [-] : Inport  Port=4
  TextureResourceID [-] : Inport  Port=5
  Bus Creator : BusCreator  Inputs='Intensity','Position','Orientation','Color','TextureResourceID'  OutDataTypeStr=Bus: PRESCAN_VISULIGHTACTUATOR_DATA  NonVirtualBus=on
  Bus Creator1 : BusCreator  Inputs=3  OutDataTypeStr=Bus: PRESCAN_RGB_DATA  NonVirtualBus=on
  Bus Creator2 : BusCreator  Inputs=3  OutDataTypeStr=Bus: PRESCAN_RPY_DATA  NonVirtualBus=on
  Bus Creator3 : BusCreator  Inputs=3  OutDataTypeStr=Bus: PRESCAN_XYZ_DATA  NonVirtualBus=on
  Data Type Conversion : DataTypeConversion  OutDataTypeStr=int32  RndMeth=Nearest
  Degrees to Radians : simulink_extras/Transformations/Degrees to Radians
  Demux : Demux  Outputs=3
  Demux1 : Demux  Outputs=3
  Demux2 : Demux  Outputs=3
  Lights : Outport
  wires:
  TextureResourceID [-]/1 -> Data Type Conversion/1  "TextureResourceID"
  MSCD [Cd]/1 -> Bus Creator/1  "Intensity"
  Bus Creator/1 -> Lights/1
  Demux/1 -> Bus Creator1/1  "R"
  Demux/2 -> Bus Creator1/2  "G"
  Demux/3 -> Bus Creator1/3  "B"
  Color [-]/1 -> Demux/1  "Color"
  Bus Creator1/1 -> Bus Creator/4  "Color"
  Demux1/1 -> Bus Creator2/1  "Roll"
  Demux1/2 -> Bus Creator2/2  "Pitch"
  Demux1/3 -> Bus Creator2/3  "Yaw"
  Orientation (RPY) [deg]/1 -> Degrees to Radians/1  "Orientation"
  Bus Creator2/1 -> Bus Creator/3  "Orientation"
  Demux2/1 -> Bus Creator3/1  "X"
  Demux2/2 -> Bus Creator3/2  "Y"
  Demux2/3 -> Bus Creator3/3  "Z"
  Position (xyz) [m]/1 -> Demux2/1  "Position"
  Bus Creator3/1 -> Bus Creator/2  "Position"
  Data Type Conversion/1 -> Bus Creator/5  "TextureResourceID"
  Degrees to Radians/1 -> Demux1/1

== system ACC_Scenario_006_cs/Mazda_RX8_1/Brake_light_right_Mux ==
  MSCD [Cd] : Inport
  Position (xyz) [m] : Inport  Port=2
  Orientation (RPY) [deg] : Inport  Port=3
  Color [-] : Inport  Port=4
  TextureResourceID [-] : Inport  Port=5
  Bus Creator : BusCreator  Inputs='Intensity','Position','Orientation','Color','TextureResourceID'  OutDataTypeStr=Bus: PRESCAN_VISULIGHTACTUATOR_DATA  NonVirtualBus=on
  Bus Creator1 : BusCreator  Inputs=3  OutDataTypeStr=Bus: PRESCAN_RGB_DATA  NonVirtualBus=on
  Bus Creator2 : BusCreator  Inputs=3  OutDataTypeStr=Bus: PRESCAN_RPY_DATA  NonVirtualBus=on
  Bus Creator3 : BusCreator  Inputs=3  OutDataTypeStr=Bus: PRESCAN_XYZ_DATA  NonVirtualBus=on
  Data Type Conversion : DataTypeConversion  OutDataTypeStr=int32  RndMeth=Nearest
  Degrees to Radians : simulink_extras/Transformations/Degrees to Radians
  Demux : Demux  Outputs=3
  Demux1 : Demux  Outputs=3
  Demux2 : Demux  Outputs=3
  Lights : Outport
  wires:
  TextureResourceID [-]/1 -> Data Type Conversion/1  "TextureResourceID"
  MSCD [Cd]/1 -> Bus Creator/1  "Intensity"
  Bus Creator/1 -> Lights/1
  Demux/1 -> Bus Creator1/1  "R"
  Demux/2 -> Bus Creator1/2  "G"
  Demux/3 -> Bus Creator1/3  "B"
  Color [-]/1 -> Demux/1  "Color"
  Bus Creator1/1 -> Bus Creator/4  "Color"
  Demux1/1 -> Bus Creator2/1  "Roll"
  Demux1/2 -> Bus Creator2/2  "Pitch"
  Demux1/3 -> Bus Creator2/3  "Yaw"
  Orientation (RPY) [deg]/1 -> Degrees to Radians/1  "Orientation"
  Bus Creator2/1 -> Bus Creator/3  "Orientation"
  Demux2/1 -> Bus Creator3/1  "X"
  Demux2/2 -> Bus Creator3/2  "Y"
  Demux2/3 -> Bus Creator3/3  "Z"
  Position (xyz) [m]/1 -> Demux2/1  "Position"
  Bus Creator3/1 -> Bus Creator/2  "Position"
  Data Type Conversion/1 -> Bus Creator/5  "TextureResourceID"
  Degrees to Radians/1 -> Demux1/1

== system ACC_Scenario_006_cs/Mazda_RX8_1/Indicator_front_left_Mux ==
  MSCD [Cd] : Inport
  Position (xyz) [m] : Inport  Port=2
  Orientation (RPY) [deg] : Inport  Port=3
  Color [-] : Inport  Port=4
  TextureResourceID [-] : Inport  Port=5
  Bus Creator : BusCreator  Inputs='Intensity','Position','Orientation','Color','TextureResourceID'  OutDataTypeStr=Bus: PRESCAN_VISULIGHTACTUATOR_DATA  NonVirtualBus=on
  Bus Creator1 : BusCreator  Inputs=3  OutDataTypeStr=Bus: PRESCAN_RGB_DATA  NonVirtualBus=on
  Bus Creator2 : BusCreator  Inputs=3  OutDataTypeStr=Bus: PRESCAN_RPY_DATA  NonVirtualBus=on
  Bus Creator3 : BusCreator  Inputs=3  OutDataTypeStr=Bus: PRESCAN_XYZ_DATA  NonVirtualBus=on
  Data Type Conversion : DataTypeConversion  OutDataTypeStr=int32  RndMeth=Nearest
  Degrees to Radians : simulink_extras/Transformations/Degrees to Radians
  Demux : Demux  Outputs=3
  Demux1 : Demux  Outputs=3
  Demux2 : Demux  Outputs=3
  Lights : Outport
  wires:
  TextureResourceID [-]/1 -> Data Type Conversion/1  "TextureResourceID"
  MSCD [Cd]/1 -> Bus Creator/1  "Intensity"
  Bus Creator/1 -> Lights/1
  Demux/1 -> Bus Creator1/1  "R"
  Demux/2 -> Bus Creator1/2  "G"
  Demux/3 -> Bus Creator1/3  "B"
  Color [-]/1 -> Demux/1  "Color"
  Bus Creator1/1 -> Bus Creator/4  "Color"
  Demux1/1 -> Bus Creator2/1  "Roll"
  Demux1/2 -> Bus Creator2/2  "Pitch"
  Demux1/3 -> Bus Creator2/3  "Yaw"
  Orientation (RPY) [deg]/1 -> Degrees to Radians/1  "Orientation"
  Bus Creator2/1 -> Bus Creator/3  "Orientation"
  Demux2/1 -> Bus Creator3/1  "X"
  Demux2/2 -> Bus Creator3/2  "Y"
  Demux2/3 -> Bus Creator3/3  "Z"
  Position (xyz) [m]/1 -> Demux2/1  "Position"
  Bus Creator3/1 -> Bus Creator/2  "Position"
  Data Type Conversion/1 -> Bus Creator/5  "TextureResourceID"
  Degrees to Radians/1 -> Demux1/1

== system ACC_Scenario_006_cs/Mazda_RX8_1/Indicator_front_right_Mux ==
  MSCD [Cd] : Inport
  Position (xyz) [m] : Inport  Port=2
  Orientation (RPY) [deg] : Inport  Port=3
  Color [-] : Inport  Port=4
  TextureResourceID [-] : Inport  Port=5
  Bus Creator : BusCreator  Inputs='Intensity','Position','Orientation','Color','TextureResourceID'  OutDataTypeStr=Bus: PRESCAN_VISULIGHTACTUATOR_DATA  NonVirtualBus=on
  Bus Creator1 : BusCreator  Inputs=3  OutDataTypeStr=Bus: PRESCAN_RGB_DATA  NonVirtualBus=on
  Bus Creator2 : BusCreator  Inputs=3  OutDataTypeStr=Bus: PRESCAN_RPY_DATA  NonVirtualBus=on
  Bus Creator3 : BusCreator  Inputs=3  OutDataTypeStr=Bus: PRESCAN_XYZ_DATA  NonVirtualBus=on
  Data Type Conversion : DataTypeConversion  OutDataTypeStr=int32  RndMeth=Nearest
  Degrees to Radians : simulink_extras/Transformations/Degrees to Radians
  Demux : Demux  Outputs=3
  Demux1 : Demux  Outputs=3
  Demux2 : Demux  Outputs=3
  Lights : Outport
  wires:
  TextureResourceID [-]/1 -> Data Type Conversion/1  "TextureResourceID"
  MSCD [Cd]/1 -> Bus Creator/1  "Intensity"
  Bus Creator/1 -> Lights/1
  Demux/1 -> Bus Creator1/1  "R"
  Demux/2 -> Bus Creator1/2  "G"
  Demux/3 -> Bus Creator1/3  "B"
  Color [-]/1 -> Demux/1  "Color"
  Bus Creator1/1 -> Bus Creator/4  "Color"
  Demux1/1 -> Bus Creator2/1  "Roll"
  Demux1/2 -> Bus Creator2/2  "Pitch"
  Demux1/3 -> Bus Creator2/3  "Yaw"
  Orientation (RPY) [deg]/1 -> Degrees to Radians/1  "Orientation"
  Bus Creator2/1 -> Bus Creator/3  "Orientation"
  Demux2/1 -> Bus Creator3/1  "X"
  Demux2/2 -> Bus Creator3/2  "Y"
  Demux2/3 -> Bus Creator3/3  "Z"
  Position (xyz) [m]/1 -> Demux2/1  "Position"
  Bus Creator3/1 -> Bus Creator/2  "Position"
  Data Type Conversion/1 -> Bus Creator/5  "TextureResourceID"
  Degrees to Radians/1 -> Demux1/1

== system ACC_Scenario_006_cs/Mazda_RX8_1/Indicator_rear_left_Mux ==
  MSCD [Cd] : Inport
  Position (xyz) [m] : Inport  Port=2
  Orientation (RPY) [deg] : Inport  Port=3
  Color [-] : Inport  Port=4
  TextureResourceID [-] : Inport  Port=5
  Bus Creator : BusCreator  Inputs='Intensity','Position','Orientation','Color','TextureResourceID'  OutDataTypeStr=Bus: PRESCAN_VISULIGHTACTUATOR_DATA  NonVirtualBus=on
  Bus Creator1 : BusCreator  Inputs=3  OutDataTypeStr=Bus: PRESCAN_RGB_DATA  NonVirtualBus=on
  Bus Creator2 : BusCreator  Inputs=3  OutDataTypeStr=Bus: PRESCAN_RPY_DATA  NonVirtualBus=on
  Bus Creator3 : BusCreator  Inputs=3  OutDataTypeStr=Bus: PRESCAN_XYZ_DATA  NonVirtualBus=on
  Data Type Conversion : DataTypeConversion  OutDataTypeStr=int32  RndMeth=Nearest
  Degrees to Radians : simulink_extras/Transformations/Degrees to Radians
  Demux : Demux  Outputs=3
  Demux1 : Demux  Outputs=3
  Demux2 : Demux  Outputs=3
  Lights : Outport
  wires:
  TextureResourceID [-]/1 -> Data Type Conversion/1  "TextureResourceID"
  MSCD [Cd]/1 -> Bus Creator/1  "Intensity"
  Bus Creator/1 -> Lights/1
  Demux/1 -> Bus Creator1/1  "R"
  Demux/2 -> Bus Creator1/2  "G"
  Demux/3 -> Bus Creator1/3  "B"
  Color [-]/1 -> Demux/1  "Color"
  Bus Creator1/1 -> Bus Creator/4  "Color"
  Demux1/1 -> Bus Creator2/1  "Roll"
  Demux1/2 -> Bus Creator2/2  "Pitch"
  Demux1/3 -> Bus Creator2/3  "Yaw"
  Orientation (RPY) [deg]/1 -> Degrees to Radians/1  "Orientation"
  Bus Creator2/1 -> Bus Creator/3  "Orientation"
  Demux2/1 -> Bus Creator3/1  "X"
  Demux2/2 -> Bus Creator3/2  "Y"
  Demux2/3 -> Bus Creator3/3  "Z"
  Position (xyz) [m]/1 -> Demux2/1  "Position"
  Bus Creator3/1 -> Bus Creator/2  "Position"
  Data Type Conversion/1 -> Bus Creator/5  "TextureResourceID"
  Degrees to Radians/1 -> Demux1/1

== system ACC_Scenario_006_cs/Mazda_RX8_1/Indicator_rear_right_Mux ==
  MSCD [Cd] : Inport
  Position (xyz) [m] : Inport  Port=2
  Orientation (RPY) [deg] : Inport  Port=3
  Color [-] : Inport  Port=4
  TextureResourceID [-] : Inport  Port=5
  Bus Creator : BusCreator  Inputs='Intensity','Position','Orientation','Color','TextureResourceID'  OutDataTypeStr=Bus: PRESCAN_VISULIGHTACTUATOR_DATA  NonVirtualBus=on
  Bus Creator1 : BusCreator  Inputs=3  OutDataTypeStr=Bus: PRESCAN_RGB_DATA  NonVirtualBus=on
  Bus Creator2 : BusCreator  Inputs=3  OutDataTypeStr=Bus: PRESCAN_RPY_DATA  NonVirtualBus=on
  Bus Creator3 : BusCreator  Inputs=3  OutDataTypeStr=Bus: PRESCAN_XYZ_DATA  NonVirtualBus=on
  Data Type Conversion : DataTypeConversion  OutDataTypeStr=int32  RndMeth=Nearest
  Degrees to Radians : simulink_extras/Transformations/Degrees to Radians
  Demux : Demux  Outputs=3
  Demux1 : Demux  Outputs=3
  Demux2 : Demux  Outputs=3
  Lights : Outport
  wires:
  TextureResourceID [-]/1 -> Data Type Conversion/1  "TextureResourceID"
  MSCD [Cd]/1 -> Bus Creator/1  "Intensity"
  Bus Creator/1 -> Lights/1
  Demux/1 -> Bus Creator1/1  "R"
  Demux/2 -> Bus Creator1/2  "G"
  Demux/3 -> Bus Creator1/3  "B"
  Color [-]/1 -> Demux/1  "Color"
  Bus Creator1/1 -> Bus Creator/4  "Color"
  Demux1/1 -> Bus Creator2/1  "Roll"
  Demux1/2 -> Bus Creator2/2  "Pitch"
  Demux1/3 -> Bus Creator2/3  "Yaw"
  Orientation (RPY) [deg]/1 -> Degrees to Radians/1  "Orientation"
  Bus Creator2/1 -> Bus Creator/3  "Orientation"
  Demux2/1 -> Bus Creator3/1  "X"
  Demux2/2 -> Bus Creator3/2  "Y"
  Demux2/3 -> Bus Creator3/3  "Z"
  Position (xyz) [m]/1 -> Demux2/1  "Position"
  Bus Creator3/1 -> Bus Creator/2  "Position"
  Data Type Conversion/1 -> Bus Creator/5  "TextureResourceID"
  Degrees to Radians/1 -> Demux1/1

== system ACC_Scenario_006_cs/Mazda_RX8_1/Indicator_side_left_Mux ==
  MSCD [Cd] : Inport
  Position (xyz) [m] : Inport  Port=2
  Orientation (RPY) [deg] : Inport  Port=3
  Color [-] : Inport  Port=4
  TextureResourceID [-] : Inport  Port=5
  Bus Creator : BusCreator  Inputs='Intensity','Position','Orientation','Color','TextureResourceID'  OutDataTypeStr=Bus: PRESCAN_VISULIGHTACTUATOR_DATA  NonVirtualBus=on
  Bus Creator1 : BusCreator  Inputs=3  OutDataTypeStr=Bus: PRESCAN_RGB_DATA  NonVirtualBus=on
  Bus Creator2 : BusCreator  Inputs=3  OutDataTypeStr=Bus: PRESCAN_RPY_DATA  NonVirtualBus=on
  Bus Creator3 : BusCreator  Inputs=3  OutDataTypeStr=Bus: PRESCAN_XYZ_DATA  NonVirtualBus=on
  Data Type Conversion : DataTypeConversion  OutDataTypeStr=int32  RndMeth=Nearest
  Degrees to Radians : simulink_extras/Transformations/Degrees to Radians
  Demux : Demux  Outputs=3
  Demux1 : Demux  Outputs=3
  Demux2 : Demux  Outputs=3
  Lights : Outport
  wires:
  TextureResourceID [-]/1 -> Data Type Conversion/1  "TextureResourceID"
  MSCD [Cd]/1 -> Bus Creator/1  "Intensity"
  Bus Creator/1 -> Lights/1
  Demux/1 -> Bus Creator1/1  "R"
  Demux/2 -> Bus Creator1/2  "G"
  Demux/3 -> Bus Creator1/3  "B"
  Color [-]/1 -> Demux/1  "Color"
  Bus Creator1/1 -> Bus Creator/4  "Color"
  Demux1/1 -> Bus Creator2/1  "Roll"
  Demux1/2 -> Bus Creator2/2  "Pitch"
  Demux1/3 -> Bus Creator2/3  "Yaw"
  Orientation (RPY) [deg]/1 -> Degrees to Radians/1  "Orientation"
  Bus Creator2/1 -> Bus Creator/3  "Orientation"
  Demux2/1 -> Bus Creator3/1  "X"
  Demux2/2 -> Bus Creator3/2  "Y"
  Demux2/3 -> Bus Creator3/3  "Z"
  Position (xyz) [m]/1 -> Demux2/1  "Position"
  Bus Creator3/1 -> Bus Creator/2  "Position"
  Data Type Conversion/1 -> Bus Creator/5  "TextureResourceID"
  Degrees to Radians/1 -> Demux1/1

== system ACC_Scenario_006_cs/Mazda_RX8_1/Indicator_side_right_Mux ==
  MSCD [Cd] : Inport
  Position (xyz) [m] : Inport  Port=2
  Orientation (RPY) [deg] : Inport  Port=3
  Color [-] : Inport  Port=4
  TextureResourceID [-] : Inport  Port=5
  Bus Creator : BusCreator  Inputs='Intensity','Position','Orientation','Color','TextureResourceID'  OutDataTypeStr=Bus: PRESCAN_VISULIGHTACTUATOR_DATA  NonVirtualBus=on
  Bus Creator1 : BusCreator  Inputs=3  OutDataTypeStr=Bus: PRESCAN_RGB_DATA  NonVirtualBus=on
  Bus Creator2 : BusCreator  Inputs=3  OutDataTypeStr=Bus: PRESCAN_RPY_DATA  NonVirtualBus=on
  Bus Creator3 : BusCreator  Inputs=3  OutDataTypeStr=Bus: PRESCAN_XYZ_DATA  NonVirtualBus=on
  Data Type Conversion : DataTypeConversion  OutDataTypeStr=int32  RndMeth=Nearest
  Degrees to Radians : simulink_extras/Transformations/Degrees to Radians
  Demux : Demux  Outputs=3
  Demux1 : Demux  Outputs=3
  Demux2 : Demux  Outputs=3
  Lights : Outport
  wires:
  TextureResourceID [-]/1 -> Data Type Conversion/1  "TextureResourceID"
  MSCD [Cd]/1 -> Bus Creator/1  "Intensity"
  Bus Creator/1 -> Lights/1
  Demux/1 -> Bus Creator1/1  "R"
  Demux/2 -> Bus Creator1/2  "G"
  Demux/3 -> Bus Creator1/3  "B"
  Color [-]/1 -> Demux/1  "Color"
  Bus Creator1/1 -> Bus Creator/4  "Color"
  Demux1/1 -> Bus Creator2/1  "Roll"
  Demux1/2 -> Bus Creator2/2  "Pitch"
  Demux1/3 -> Bus Creator2/3  "Yaw"
  Orientation (RPY) [deg]/1 -> Degrees to Radians/1  "Orientation"
  Bus Creator2/1 -> Bus Creator/3  "Orientation"
  Demux2/1 -> Bus Creator3/1  "X"
  Demux2/2 -> Bus Creator3/2  "Y"
  Demux2/3 -> Bus Creator3/3  "Z"
  Position (xyz) [m]/1 -> Demux2/1  "Position"
  Bus Creator3/1 -> Bus Creator/2  "Position"
  Data Type Conversion/1 -> Bus Creator/5  "TextureResourceID"
  Degrees to Radians/1 -> Demux1/1

== system ACC_Scenario_006_cs/Mazda_RX8_1/JointGroup_WheelDisplacement_V2R ==
  Velocity [m/s] : Inport  SampleTime=TimeStep
  Discrete-Time Integrator : DiscreteIntegrator  SampleTime=TimeStep
  omega=V/Rwheel : Gain  Gain=1/TireRadius
  Rotation [rad] : Outport
  wires:
  Discrete-Time Integrator/1 -> Rotation [rad]/1  "roty"
  omega=V/Rwheel/1 -> Discrete-Time Integrator/1  "rotational speed [rad/s]"
  Velocity [m/s]/1 -> omega=V/Rwheel/1

== system ACC_Scenario_006_cs/Mazda_RX8_1/SELF_Demux ==
  SELF : Inport  OutDataTypeStr=Bus: PRESCAN_SELFSENSORDATA
  Bus Selector : BusSelector  OutputSignals=PositionX,PositionY,PositionZ,OrientationRoll,OrientationPitch,OrientationYaw,Velocity,Yaw_rate,Lat,Long,Alt
  Demux2 : Demux  Outputs=3
  Gain : Gain  Gain=180/pi
  Gain1 : Gain  Gain=180/pi
  Vector Concatenate1 : Concatenate  NumInputs=3
  compas converter : Subsystem
  x [m] : Outport
  y [m] : Outport  Port=2
  z [m] : Outport  Port=3
  rotx [deg] : Outport  Port=4
  roty [deg] : Outport  Port=5
  rotz [deg] : Outport  Port=6
  GPS lat [deg] : Outport  Port=7
  GPS long [deg] : Outport  Port=8
  GPS alt [m] : Outport  Port=9
  velocity [m/s] : Outport  Port=10
  heading [deg] : Outport  Port=11
  yaw rate [deg/s] : Outport  Port=12
  wires:
  Bus Selector/11 -> GPS alt [m]/1  "<Alt>"
  Bus Selector/10 -> GPS long [deg]/1  "<Long>"
  Bus Selector/9 -> GPS lat [deg]/1  "<Lat>"
  Bus Selector/8 -> Gain1/1  "<Yaw_rate>"
  Bus Selector/7 -> velocity [m/s]/1  "<Velocity>"
  Bus Selector/6 -> compas converter/1(rotz [rad]), Vector Concatenate1/3  "<OrientationYaw>"
  Bus Selector/5 -> Vector Concatenate1/2  "<OrientationPitch>"
  Bus Selector/4 -> Vector Concatenate1/1  "<OrientationRoll>"
  Vector Concatenate1/1 -> Gain/1
  Bus Selector/3 -> z [m]/1  "<PositionZ>"
  Bus Selector/2 -> y [m]/1  "<PositionY>"
  Bus Selector/1 -> x [m]/1  "<PositionX>"
  SELF/1 -> Bus Selector/1
  Gain/1 -> Demux2/1
  Demux2/1 -> rotx [deg]/1
  Demux2/2 -> roty [deg]/1
  Demux2/3 -> rotz [deg]/1
  compas converter/1(heading [deg]) -> heading [deg]/1
  Gain1/1 -> yaw rate [deg/s]/1
